simulink model "AFCSModel"  (R2025b)
settings: Solver=ode4  StartTime=0.0  StopTime=200  FixedStep=0.01  RelTol=1e-3  EnableMultiTasking=on
values from neighbouring files (symbols this model uses):
  AD = [0.05526	0.05526	0.05568	0.05804	0.06460	0.08210 ... (first row only)    [AirCraftData.m]
  Alpha0 = [0.143	0.143	0.122	-0.267	-0.627	0.120 ... (first row only)    [AirCraftData.m]
  alt = 1284.73    [Start.m]    (also in drl_simplified_dynamics.m)
  CA = 3.451    [AirCraftData.m]    (also in AircraftTrim.m)
  CDmin = [0.03799	0.03799	0.03799	0.03799	0.03904	0.04277 ... (first row only)    [AirCraftData.m]
  CLAlpha = [0.1012	0.1021	0.1033	0.1051	0.1079	0.0976 ... (first row only)    [AirCraftData.m]
  Clbt0 = [-0.00147	-0.00148	-0.00149	-0.00153	-0.00158	-0.00171 ... (first row only)    [AirCraftData.m]
  Clbtaf = [0	0	0	0	0	0;0	 0	0	0	0	0]    [AirCraftData.m]
  ClDelA = [-0.003110	-0.003065	-0.003040	-0.003036	-0.003052	-0.003088 ... (first row only)    [AirCraftData.m]
  CLDelE = [0.00653	0.00668	0.00690	0.00724	0.00772	0.00846 ... (first row only)    [AirCraftData.m]
  ClDelR = [0.000584	0.000605	0.000638	0.000686	0.000760	0.000877 ... (first row only)    [AirCraftData.m]
  CLDM = [0.244	0.244	0.244	0.244	0.244	0.244 ... (first row only)    [AirCraftData.m]
  Clp0 = [-0.5510 	-0.5610 	-0.5767 	-0.6005 	-0.6224 	-0.6763 ... (first row only)    [AirCraftData.m]
  ClpAf = [0,0,0,0,0,0;0,0,0,0,0,0]    [AirCraftData.m]
  Clr0 = [0.1308 	0.1339 	0.1383 	0.1474 	0.1601 	0.1738 ... (first row only)    [AirCraftData.m]
  ClrAf = [0,0,0,0,0,0;0,0,0,0,0,0]    [AirCraftData.m]
  Cm0 = [0.2014	0.2017	0.2034	0.2083	0.2207	0.2475 ... (first row only)    [AirCraftData.m]
  CmAfdot = [-11.5890 	-12.0169 	-12.7558 	-13.8010 	-15.2088 	-16.2278 ... (first row only)    [AirCraftData.m]
  CmCl = [-0.3454	-0.3441	-0.3427	-0.3412	-0.3396	-0.3379 ... (first row only)    [AirCraftData.m]
  CmDelE = [-0.03554	-0.03651	-0.03802	-0.04028	-0.04365	-0.04798 ... (first row only)    [AirCraftData.m]
  Cmq0 = [-42.0260 	-42.2665 	-42.9499 	-44.8315 	-45.5877 	-46.0842 ... (first row only)    [AirCraftData.m]
  CN1A0 = [0.0740	0.0662	0.0605	0.0552	0.0554 ... (first row only)    [AirCraftData.m]
  Cnbt0 = [0.00180	0.00183	0.00187	0.00192	0.00200	0.00207 ... (first row only)    [AirCraftData.m]
  Cnbtaf = [-0.000030 	-0.000031 	-0.000031 	-0.000032 	-0.000033 	-0.000035 ... (first row only)    [AirCraftData.m]
  CnDelA0 = [-0.000180	-0.000178	-0.000176	-0.000176	-0.000177	-0.000179 ... (first row only)    [AirCraftData.m]
  CnDelAAf = [0	 0	0	0	0	0;0	 0	0	0	0	0]    [AirCraftData.m]
  CnDelR = [-0.002214	-0.002274	-0.002367	-0.002505	-0.002712	-0.003039 ... (first row only)    [AirCraftData.m]
  Cnp0 = [0.0521 	0.0532 	0.0571 	0.0601 	0.0636 	0.0664 ... (first row only)    [AirCraftData.m]
  CnpAf = [0,0,0,0,0,0;0,0,0,0,0,0]    [AirCraftData.m]
  Cnr = [-0.1810 	-0.1832 	-0.1855 	-0.1892 	-0.1933 	-0.1973 ... (first row only)    [AirCraftData.m]
  Cxh_Slip = [0.0000, 0.0045, 0.0089, 0.0132, 0.0174 ... (first row only)    [AirCraftData.m]
  Cybeta0 = [-0.01783	-0.01790	-0.01804	-0.01824	-0.01851	-0.01884 ... (first row only)    [AirCraftData.m]
  Cybtaf = [0 0 0 0 0 0;0 0 0 0 0 0]    [AirCraftData.m]
  CyDelA = [0.000287	0.000295	0.000307	0.000325	0.000351	0.000394 ... (first row only)    [AirCraftData.m]
  CyDelR = [0.004946	0.005035	0.005316	0.005791	0.006458	0.007318 ... (first row only)    [AirCraftData.m]
  Cyh_Slip = [0.0000, -0.0248, -0.0519, -0.0813, -0.1130 ... (first row only)    [AirCraftData.m]
  ETA_data = [0.729 0.727 0.72 0.71 0.877 0.858 0.855 0.853 0.857 0.862 0.87 0.796 ... (330 elements, 11x5x6)]    [ETA_data.mat]
  eul_0 = [0/57.3 0/57.3 0/57.3]    [AircraftTrim.m]
  F = A(:, 1)    [drl_simplified_dynamics.m]    (also in func_DrawAircraftModel.m = [         1,  2,  3,  1;         1,  3,  4,  1;         1,  )
  flap = 0    [AircraftTrim.m]
  inertia = [  Ix      Iy     Iz  Ixz]    [AircraftTrim.m]
  Initi_Heading = 15.95*pi/180    (= 0.278380015693)    [Start.m]
  Initi_Lati = 32.6261    [Start.m]
  Initi_Longi = 103.5940    (= 103.594)    [Start.m]
  mass = 54000    [Start.m]    (also in drl_simplified_dynamics.m)
  op = evalin('base', 'op')    [drl_simplified_dynamics.m]
  q = func_GreatCircleForward(start_lat, start_lon, leg_bearing, local_s)    [system_model_update.m]
  r = r1 + r2    [drl_piecewise_reward.m]    (also in drl_reward_function.m)
  RNPAR_FlightPlan = JiuZhaiHuangLong_RNPAR_FlightPlan    [Manuscript_RNPAR_FlightPlan.m]
  Vab_0 = [Vt 0 0]    [AircraftTrim.m]
  Vt = 80    [Start.m]    (also in drl_simplified_dynamics.m; setup_afcs_system_model_test.m)
  wind_direction = 0    [Start.m]
  wind_type = 2    [Start.m]
  Wxyz_0 = [0 0 0]    [AircraftTrim.m]
  X = 1.06    [AircraftTrim.m]
  xme_0 = [0 0 -alt]    [AircraftTrim.m]
  Y = 1.177    [AircraftTrim.m]
undefined symbols (not defined in the file or in its folder): func_SystemModelMonitorBlock, Light, MIL, slselsubs, thrust_data
libraries: simulink_extras x4, aerolibatmos2 x3, aerolibconvert2 x3, aerolibwind2 x3, sharedutil x2, aerolibobsolete x1
(part 2 of 3)

== system AFCSModel/Plane&Actuator/PlaneModel/Aero Moment ==
  note: L
  note: M
  note: N
  V Alpha Beta : Inport
  QS : Inport  Port=2
  delta_a delta_e delta_r : Inport  Port=3
  p q r : Inport  Port=4
  delta_p : Inport  Port=5
  Thrust : Inport  Port=6
  delta_flap : Inport  Port=7
  Calculate Roll Moment L : Subsystem
  Calculate Yaw Moment N : Subsystem
  Calculate pitch Moment M : Subsystem
  Mux2 : Mux  Inputs=3
  Ma_b : Outport
  wires:
  Mux2/1 -> Ma_b/1
  QS/1 -> Calculate Roll Moment L/2(QS), Calculate pitch Moment M/1(QS), Calculate Yaw Moment N/2(QS)
  V Alpha Beta/1 -> Calculate Roll Moment L/1(V Alpha Beta), Calculate pitch Moment M/2(V alpha beta), Calculate Yaw Moment N/1(V Alpha Beta)
  delta_p/1 -> Calculate pitch Moment M/3(delta_p), Calculate Roll Moment L/5(delta_p), Calculate Yaw Moment N/5(delta_p)
  delta_a delta_e delta_r/1 -> Calculate Roll Moment L/3(delta_a delta_e delta_r), Calculate pitch Moment M/4(delta_a delta_e delta_r), Calculate Yaw Moment N/3(delta_a delta_e delta_r)
  p q r/1 -> Calculate Roll Moment L/4(p q r), Calculate pitch Moment M/5(p q r), Calculate Yaw Moment N/4(p q r)
  Calculate pitch Moment M/1(M) -> Mux2/2
  Calculate Roll Moment L/1(L) -> Mux2/1
  Calculate Yaw Moment N/1(N) -> Mux2/3
  Thrust/1 -> Calculate pitch Moment M/6(Thrust), Calculate Roll Moment L/6(Thrust)
  delta_flap/1 -> Calculate Roll Moment L/7(delta_flap), Calculate pitch Moment M/7(delta_flap), Calculate Yaw Moment N/6(delta_flap)

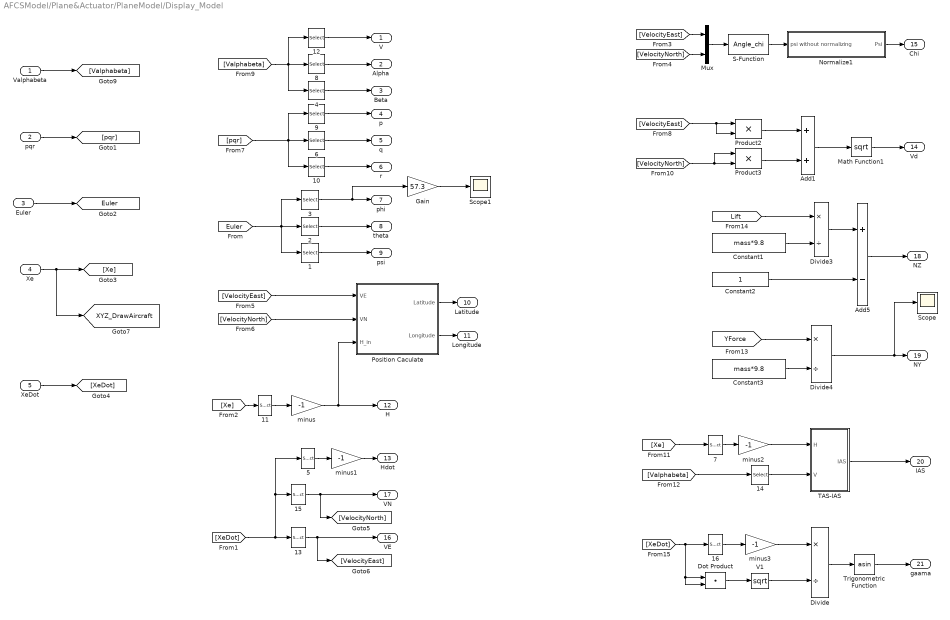
== system AFCSModel/Plane&Actuator/PlaneModel/Display_Model ==
  Valphabeta : Inport
  pqr : Inport  Port=2
  Euler : Inport  Port=3
  Xe : Inport  Port=4
  XeDot : Inport  Port=5
  {1,4..5,7,10..11,16} (7 alike) : Selector  InputPortWidth=3  IndexOptions=Index vector (dialog)  Indices=3  OutputSizes=[(-2)]
  {3,9,12,14..15} (5 alike) : Selector  InputPortWidth=3  IndexOptions=Index vector (dialog)  Indices=1  OutputSizes=[(-2)]
  {2,6,8,13} (4 alike) : Selector  InputPortWidth=3  IndexOptions=Index vector (dialog)  Indices=2  OutputSizes=[(-2)]
  Add1 : Sum
  Add5 : Sum  Inputs=+-
  Constant1 : Constant  Value=mass*9.8
  Constant2 : Constant
  Constant3 : Constant  Value=mass*9.8
  Divide : Product  Inputs=*/
  Divide3 : Product  Inputs=*/
  Divide4 : Product  Inputs=*/
  Dot Product : DotProduct  SaturateOnIntegerOverflow=on  InputSameDT=off  OutDataTypeStr=Inherit: Inherit via internal rule
  Gain : Gain  Gain=57.3
  Math Function1 : Math  Operator=sqrt  SignedPower=on
  Mux : Mux  Inputs=2
  Normalize1 : Subsystem
  Position Caculate : Subsystem
  Product2 : Product  RndMeth=Zero
  Product3 : Product  RndMeth=Zero
  S-Function : S-Function  FunctionName=Angle_chi  SFunctionDeploymentMode=off  EnableBusSupport=off
  Scope : Scope
      settings: ActiveDisplayYMinimum=-0.01745  ActiveDisplayYMaximum=0.03101  DataLoggingVariableName=ScopeData3
  Scope1 : Scope
      settings: ActiveDisplayYMinimum=-1.2868572992970082  ActiveDisplayYMaximum=11.581951961084815
  TAS-IAS : Subsystem
  Trigonometric Function : Trigonometry  Operator=asin
  V1 : Math  Operator=sqrt  SignedPower=on
  minus{,1..3} (4 alike) : Gain  Gain=-1
  V : Outport
  Alpha : Outport  Port=2
  Beta : Outport  Port=3
  p : Outport  Port=4
  q : Outport  Port=5
  r : Outport  Port=6
  phi : Outport  Port=7
  theta : Outport  Port=8
  psi : Outport  Port=9
  Latitude : Outport  Port=10
  Longitude : Outport  Port=11
  H : Outport  Port=12
  Hdot : Outport  Port=13
  Vd : Outport  Port=14
  Chi : Outport  Port=15
  VE : Outport  Port=16
  VN : Outport  Port=17
  NZ : Outport  Port=18
  NY : Outport  Port=19
  IAS : Outport  Port=20
  gaama : Outport  Port=21
  tag scope: Euler=global, XYZ_DrawAircraft=global
  wires:
  [Xe] -> 11/1
  11/1 -> minus/1
  [pqr] -> 6/1, 9/1, 10/1
  [Euler] -> 2/1, 3/1, 1/1
  [Valphabeta] -> 8/1, 12/1, 4/1
  12/1 -> V/1
  Valphabeta/1 -> [Valphabeta]
  pqr/1 -> [pqr]
  Euler/1 -> [Euler]
  Xe/1 -> [XYZ_DrawAircraft], [Xe]
  [XeDot] -> 15/1, 5/1, 13/1
  5/1 -> minus1/1
  13/1 -> [VelocityEast], VE/1
  minus1/1 -> Hdot/1
  XeDot/1 -> [XeDot]
  15/1 -> [VelocityNorth], VN/1
  S-Function/1 -> Normalize1/1(psi without normalizing)
  Normalize1/1(Psi) -> Chi/1
  Mux/1 -> S-Function/1
  [VelocityEast] -> Mux/1
  [VelocityNorth] -> Mux/2
  [VelocityEast] -> Position Caculate/1(VE)
  [VelocityNorth] -> Position Caculate/2(VN)
  Position Caculate/1(Latitude) -> Latitude/1
  Position Caculate/2(Longitude) -> Longitude/1
  Product2/1 -> Add1/1
  Product3/1 -> Add1/2
  Math Function1/1 -> Vd/1
  Add1/1 -> Math Function1/1
  [VelocityNorth] -> Product3/1, Product3/2
  [VelocityEast] -> Product2/2, Product2/1
  [Xe] -> 7/1
  7/1 -> minus2/1
  minus2/1 -> TAS-IAS/1(H)
  minus/1 -> Position Caculate/3(H_in), H/1
  [Valphabeta] -> 14/1
  14/1 -> TAS-IAS/2(V)
  TAS-IAS/1(IAS) -> IAS/1
  Divide4/1 -> Scope/1, NY/1
  Constant3/1 -> Divide4/2
  [YForce] -> Divide4/1
  [Lift] -> Divide3/1
  Constant1/1 -> Divide3/2
  Divide3/1 -> Add5/1
  Constant2/1 -> Add5/2
  Add5/1 -> NZ/1
  1/1 -> psi/1
  2/1 -> theta/1
  3/1 -> Gain/1, phi/1
  10/1 -> r/1
  6/1 -> q/1
  9/1 -> p/1
  4/1 -> Beta/1
  8/1 -> Alpha/1
  Trigonometric Function/1 -> gaama/1
  Divide/1 -> Trigonometric Function/1
  16/1 -> minus3/1
  [XeDot] -> Dot Product/2, Dot Product/1, 16/1
  Dot Product/1 -> V1/1
  minus3/1 -> Divide/1
  V1/1 -> Divide/2
  Gain/1 -> Scope1/1

== system AFCSModel/Plane&Actuator/PlaneModel/Engine ==
  Alt : Inport
  V : Inport  Port=2
  delta_p : Inport  Port=3
  Calculate Force : Lookup_n-D  NumberOfTableDimensions=3  BreakpointsForDimension1=[0,1000,2000,3000,4000,5000,6000,7000,8000,9000,10000]  BreakpointsForDimension2=[50,100,150,175,200]  BreakpointsForDimension3=[0.2,0.4,0.6,0.7,0.85,1,1.04]  BreakpointsForDimension5=slselsubs({[1:3], [1:3], [1:3], [1:3], [1:3], [1:3], [1:3], [1:3], [1:3], [1:3], [1:3], [1:3], [1:3], [1:3], [1:3], [1:3], [1:3], [1:3], [1:3], [1:3], [1:3], [1:3], [1:3], [1:3], [1:3], [1:3]}, 1)  BreakpointsForDimension6=slselsubs({[1:3], [1:3], [1:3], [1:3], [1:3], [1:3], [1:3], [1:3], [1:3], [1:3], [1:3], [1:3], [1:3], [1:3], [1:3], [1:3], [1:3], [1:3], [1:3], [1:3], [1:3], [1:3], [1:3], [1:3], [1:3], [1:3]}, 2)  BreakpointsForDimension7=slselsubs({[1:3], [1:3], [1:3], [1:3], [1:3], [1:3], [1:3], [1:3], [1:3], [1:3], [1:3], [1:3], [1:3], [1:3], [1:3], [1:3], [1:3], [1:3], [1:3], [1:3], [1:3], [1:3], [1:3], [1:3], [1:3], [1:3]}, 3)  BreakpointsForDimension8=slselsubs({[1:3], [1:3], [1:3], [1:3], [1:3], [1:3], [1:3], [1:3], [1:3], [1:3], [1:3], [1:3], [1:3], [1:3], [1:3], [1:3], [1:3], [1:3], [1:3], [1:3], [1:3], [1:3], [1:3], [1:3], [1:3], [1:3]}, 4)  BreakpointsForDimension9=slselsubs({[1:3], [1:3], [1:3], [1:3], [1:3], [1:3], [1:3], [1:3], [1:3], [1:3], [1:3], [1:3], [1:3], [1:3], [1:3], [1:3], [1:3], [1:3], [1:3], [1:3], [1:3], [1:3], [1:3], [1:3], [1:3], [1:3]}, 5)  BreakpointsForDimension10=slselsubs({[1:3], [1:3], [1:3], [1:3], [1:3], [1:3], [1:3], [1:3], [1:3], [1:3], [1:3], [1:3], [1:3], [1:3], [1:3], [1:3], [1:3], [1:3], [1:3], [1:3], [1:3], [1:3], [1:3], [1:3], [1:3], [1:3]}, 6)  BreakpointsForDimension11=slselsubs({[1:3], [1:3], [1:3], [1:3], [1:3], [1:3], [1:3], [1:3], [1:3], [1:3], [1:3], [1:3], [1:3], [1:3], [1:3], [1:3], [1:3], [1:3], [1:3], [1:3], [1:3], [1:3], [1:3], [1:3], [1:3], [1:3]}, 7)  BreakpointsForDimension12=slselsubs({[1:3], [1:3], [1:3], [1:3], [1:3], [1:3], [1:3], [1:3], [1:3], [1:3], [1:3], [1:3], [1:3], [1:3], [1:3], [1:3], [1:3], [1:3], [1:3], [1:3], [1:3], [1:3], [1:3], [1:3], [1:3], [1:3]}, 8)  BreakpointsForDimension13=slselsubs({[1:3], [1:3], [1:3], [1:3], [1:3], [1:3], [1:3], [1:3], [1:3], [1:3], [1:3], [1:3], [1:3], [1:3], [1:3], [1:3], [1:3], [1:3], [1:3], [1:3], [1:3], [1:3], [1:3], [1:3], [1:3], [1:3]}, 9)  BreakpointsForDimension14=slselsubs({[1:3], [1:3], [1:3], [1:3], [1:3], [1:3], [1:3], [1:3], [1:3], [1:3], [1:3], [1:3], [1:3], [1:3], [1:3], [1:3], [1:3], [1:3], [1:3], [1:3], [1:3], [1:3], [1:3], [1:3], [1:3], [1:3]}, 10)  BreakpointsForDimension15=slselsubs({[1:3], [1:3], [1:3], [1:3], [1:3], [1:3], [1:3], [1:3], [1:3], [1:3], [1:3], [1:3], [1:3], [1:3], [1:3], [1:3], [1:3], [1:3], [1:3], [1:3], [1:3], [1:3], [1:3], [1:3], [1:3], [1:3]}, 11)  BreakpointsForDimension16=slselsubs({[1:3], [1:3], [1:3], [1:3], [1:3], [1:3], [1:3], [1:3], [1:3], [1:3], [1:3], [1:3], [1:3], [1:3], [1:3], [1:3], [1:3], [1:3], [1:3], [1:3], [1:3], [1:3], [1:3], [1:3], [1:3], [1:3]}, 12)  BreakpointsForDimension17=slselsubs({[1:3], [1:3], [1:3], [1:3], [1:3], [1:3], [1:3], [1:3], [1:3], [1:3], [1:3], [1:3], [1:3], [1:3], [1:3], [1:3], [1:3], [1:3], [1:3], [1:3], [1:3], [1:3], [1:3], [1:3], [1:3], [1:3]}, 13)  BreakpointsForDimension18=slselsubs({[1:3], [1:3], [1:3], [1:3], [1:3], [1:3], [1:3], [1:3], [1:3], [1:3], [1:3], [1:3], [1:3], [1:3], [1:3], [1:3], [1:3], [1:3], [1:3], [1:3], [1:3], [1:3], [1:3], [1:3], [1:3], [1:3]}, 14)  BreakpointsForDimension19=slselsubs({[1:3], [1:3], [1:3], [1:3], [1:3], [1:3], [1:3], [1:3], [1:3], [1:3], [1:3], [1:3], [1:3], [1:3], [1:3], [1:3], [1:3], [1:3], [1:3], [1:3], [1:3], [1:3], [1:3], [1:3], [1:3], [1:3]}, 15)  BreakpointsForDimension20=slselsubs({[1:3], [1:3], [1:3], [1:3], [1:3], [1:3], [1:3], [1:3], [1:3], [1:3], [1:3], [1:3], [1:3], [1:3], [1:3], [1:3], [1:3], [1:3], [1:3], [1:3], [1:3], [1:3], [1:3], [1:3], [1:3], [1:3]}, 16)  BreakpointsForDimension21=slselsubs({[1:3], [1:3], [1:3], [1:3], [1:3], [1:3], [1:3], [1:3], [1:3], [1:3], [1:3], [1:3], [1:3], [1:3], [1:3], [1:3], [1:3], [1:3], [1:3], [1:3], [1:3], [1:3], [1:3], [1:3], [1:3], [1:3]}, 17)  BreakpointsForDimension22=slselsubs({[1:3], [1:3], [1:3], [1:3], [1:3], [1:3], [1:3], [1:3], [1:3], [1:3], [1:3], [1:3], [1:3], [1:3], [1:3], [1:3], [1:3], [1:3], [1:3], [1:3], [1:3], [1:3], [1:3], [1:3], [1:3], [1:3]}, 18)  BreakpointsForDimension23=slselsubs({[1:3], [1:3], [1:3], [1:3], [1:3], [1:3], [1:3], [1:3], [1:3], [1:3], [1:3], [1:3], [1:3], [1:3], [1:3], [1:3], [1:3], [1:3], [1:3], [1:3], [1:3], [1:3], [1:3], [1:3], [1:3], [1:3]}, 19)  BreakpointsForDimension24=slselsubs({[1:3], [1:3], [1:3], [1:3], [1:3], [1:3], [1:3], [1:3], [1:3], [1:3], [1:3], [1:3], [1:3], [1:3], [1:3], [1:3], [1:3], [1:3], [1:3], [1:3], [1:3], [1:3], [1:3], [1:3], [1:3], [1:3]}, 20)  BreakpointsForDimension25=slselsubs({[1:3], [1:3], [1:3], [1:3], [1:3], [1:3], [1:3], [1:3], [1:3], [1:3], [1:3], [1:3], [1:3], [1:3], [1:3], [1:3], [1:3], [1:3], [1:3], [1:3], [1:3], [1:3], [1:3], [1:3], [1:3], [1:3]}, 21)  BreakpointsForDimension26=slselsubs({[1:3], [1:3], [1:3], [1:3], [1:3], [1:3], [1:3], [1:3], [1:3], [1:3], [1:3], [1:3], [1:3], [1:3], [1:3], [1:3], [1:3], [1:3], [1:3], [1:3], [1:3], [1:3], [1:3], [1:3], [1:3], [1:3]}, 22)  BreakpointsForDimension27=slselsubs({[1:3], [1:3], [1:3], [1:3], [1:3], [1:3], [1:3], [1:3], [1:3], [1:3], [1:3], [1:3], [1:3], [1:3], [1:3], [1:3], [1:3], [1:3], [1:3], [1:3], [1:3], [1:3], [1:3], [1:3], [1:3], [1:3]}, 23)  BreakpointsForDimension28=slselsubs({[1:3], [1:3], [1:3], [1:3], [1:3], [1:3], [1:3], [1:3], [1:3], [1:3], [1:3], [1:3], [1:3], [1:3], [1:3], [1:3], [1:3], [1:3], [1:3], [1:3], [1:3], [1:3], [1:3], [1:3], [1:3], [1:3]}, 24)  BreakpointsForDimension29=slselsubs({[1:3], [1:3], [1:3], [1:3], [1:3], [1:3], [1:3], [1:3], [1:3], [1:3], [1:3], [1:3], [1:3], [1:3], [1:3], [1:3], [1:3], [1:3], [1:3], [1:3], [1:3], [1:3], [1:3], [1:3], [1:3], [1:3]}, 25)  BreakpointsForDimension30=slselsubs({[1:3], [1:3], [1:3], [1:3], [1:3], [1:3], [1:3], [1:3], [1:3], [1:3], [1:3], [1:3], [1:3], [1:3], [1:3], [1:3], [1:3], [1:3], [1:3], [1:3], [1:3], [1:3], [1:3], [1:3], [1:3], [1:3]}, 26)  Table=thrust_data  InterpMethod=Cubic spline  ExtrapMethod=Cubic spline
      settings: InputPortMap=u0,u1,u2
  Thrust : Outport
  wires:
  Calculate Force/1 -> Thrust/1
  delta_p/1 -> Calculate Force/3
  Alt/1 -> Calculate Force/1
  V/1 -> Calculate Force/2

== system AFCSModel/Plane&Actuator/PlaneModel/ISA ==
  note: V
  note: V^2
  V : Inport
  Alt : Inport  Port=2
  Constant2 : Constant  Value=0.5
  Divide : Product  Inputs=/*
  ISA Atmosphere Model : aerolibatmos2/ISA Atmosphere Model  useExtended=off  action=Warning  custom=off  viscosityOut=off  g=9.80665  gamma=1.4  R=287.0531  L=0.0065  h_trop=11000  h_strat=20000  rho0=1.225  P0=101325  T0=288.15  h0=0  S=110.4  Tref=273.15  muref=1.716e-5
  Product : Product  Inputs=3  RndMeth=Zero
  Product2 : Product  RndMeth=Zero
  Scope1 : Scope
  Scope2 : Scope
      settings: DataLoggingVariableName=ScopeData2
  To Workspace : ToWorkspace  VariableName=Rou  SampleTime=-1
  Qs : Outport
  tag scope: Alt=global, Ma=global
  wires:
  ISA Atmosphere Model/4 -> To Workspace/1, Product/1
  Alt/1 -> ISA Atmosphere Model/1, [Alt]
  ISA Atmosphere Model/1 -> Scope2/1
  ISA Atmosphere Model/3 -> Scope1/1
  Product/1 -> Qs/1
  Divide/1 -> [Ma]
  ISA Atmosphere Model/2 -> Divide/1
  Product2/1 -> Product/3
  Constant2/1 -> Product/2
  V/1 -> Divide/2, Product2/1, Product2/2

== system AFCSModel/Plane&Actuator/PlaneModel/RusPlane ==
  Force : Inport
  Moment : Inport  Port=2
  AV Alpha Beta : Subsystem
  AV Alpha Beta_Trans : Subsystem
  BWxyz2 : Integrator  InitialCondition=op.States(2).x
  Calculate DCM & Euler Angles : Subsystem  AncestorBlock=aerolib6dofsys/DCM & Euler Angles (Euler)  mask(DCM & Euler Angles (Euler)){}
  Constant1 : Constant  Value=inertia  OutDataTypeStr=Inherit: Inherit via back propagation
  Constant2 : Constant  Value=mass  OutDataTypeStr=Inherit: Inherit via back propagation
  Product : Product  Inputs=*/  SaturateOnIntegerOverflow=on  OutDataTypeStr=Inherit: Same as first input
  Subsystem : Subsystem
  Subsystem1 : Subsystem
  Sum : Sum  Inputs=|++  SaturateOnIntegerOverflow=on
  Vbxw : sharedutil/3x3 Cross Product  aMode=aMode
      settings: LibrarySourceBlock=aerolibutil/3x3 Cross Product
  xe,ye,ze : Integrator  InitialCondition=op.States(4).x
  V alpha beta : Outport
  p q r : Outport  Port=2
  Euler : Outport  Port=3
  Xe : Outport  Port=4
  XeDot : Outport  Port=5
  tag scope: Plane_uvw=global
  wires:
  Constant1/1 -> Subsystem/3(inertia Ix Iy Iz Ixz)
  Product/1 -> Sum/1
  Sum/1 -> AV Alpha Beta/1(udot vdot wdot)
  Vbxw/1 -> Sum/2
  Constant2/1 -> Product/2
  BWxyz2/1 -> Calculate DCM & Euler Angles/1("Wxyz "), p q r/1, Vbxw/2, Subsystem/2(pqr)  "pqr"
  Subsystem1/1(Xedot Yedot Zedot) -> XeDot/1, xe,ye,ze/1
  Force/1 -> Product/1  "Force"
  xe,ye,ze/1 -> Xe/1  "Xe"
  Calculate DCM & Euler Angles/1(Euler) -> Euler/1, Subsystem1/2(Euler phi theta psi)  "Eular"
  AV Alpha Beta/2(u v w in) -> Vbxw/1, [Plane_uvw], Subsystem1/1("U V W ")
  AV Alpha Beta/1(V alpha beta) -> AV Alpha Beta_Trans/1(V alpha beta input)
  Subsystem/1(pdot qdot rdot) -> BWxyz2/1
  Moment/1 -> Subsystem/1(Moment L M N)  "Moment"
  AV Alpha Beta_Trans/1(Valphabeta) -> V alpha beta/1

== system AFCSModel/RNP AR Approach Guidance/L1GuidanceVersion1/Subsystem ==
  YZ : Inport
  Lfw : Inport  Port=2
  eta1 : Inport  Port=3
  R_turn : Inport  Port=4
  turnDir : Inport  Port=5
  legType : Inport  Port=6
  Divide : Product  Inputs=*/
  Gain : Gain  Gain=-1
  Plus : Sum
  Scope : Scope
      settings: ActiveDisplayYMinimum=-1  ActiveDisplayYMaximum=1  DataLoggingVariableName=ScopeData9
  Scope1 : Scope
      settings: ActiveDisplayYMinimum=-1  ActiveDisplayYMaximum=1  DataLoggingVariableName=ScopeData10
  Square : Math  Operator=square
  Square1 : Math  Operator=square
  caculateL1 : Sqrt
  eta2TF : Trigonometry  Operator=atan
  etaTF : Sum
  L1 : Outport
  eta : Outport  Port=2
  wires:
  Square1/1 -> Plus/2
  Square/1 -> Plus/1
  Plus/1 -> caculateL1/1
  YZ/1 -> Square/1, Divide/1
  Lfw/1 -> Square1/1, Divide/2
  Divide/1 -> eta2TF/1
  eta1/1 -> Gain/1
  eta2TF/1 -> etaTF/2, Scope1/1
  etaTF/1 -> eta/1
  Gain/1 -> Scope/1, etaTF/1
  caculateL1/1 -> L1/1

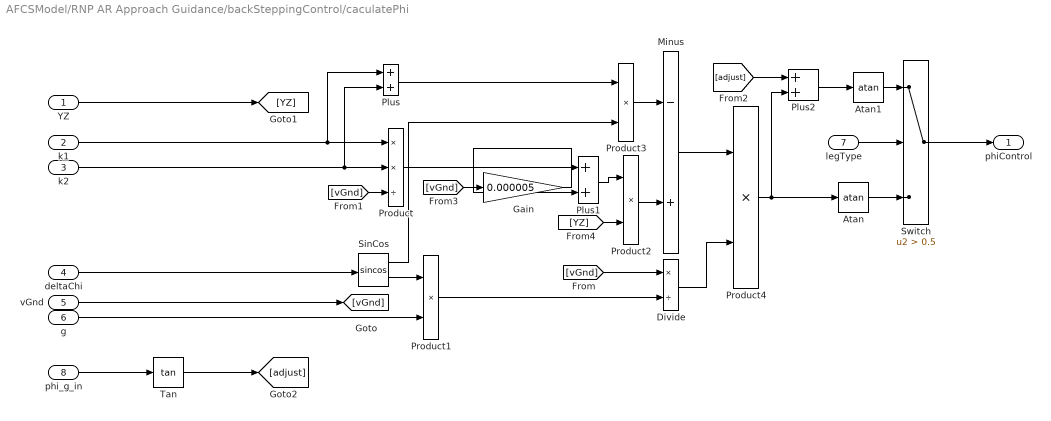
== system AFCSModel/RNP AR Approach Guidance/backSteppingControl/caculatePhi ==
  YZ : Inport
  k1 : Inport  Port=2
  k2 : Inport  Port=3
  deltaChi : Inport  Port=4
  vGnd : Inport  Port=5
  g : Inport  Port=6
  legType : Inport  Port=7
  phi_g_in : Inport  Port=8
  Atan : Trigonometry  Operator=atan
  Atan1 : Trigonometry  Operator=atan
  Divide : Product  Inputs=*/
  Gain : Gain  Gain=0.000005
  Minus : Sum  Inputs=-+
  Plus : Sum
  Plus1 : Sum
  Plus2 : Sum
  Product : Product  Inputs=**/
  Product{1..4} (4 alike) : Product
  SinCos : Trigonometry  Operator=sincos
  Switch : Switch  Criteria=u2 > Threshold  Threshold=0.5  SaturateOnIntegerOverflow=off  InputSameDT=off
  Tan : Trigonometry  Operator=tan
  phiControl : Outport
  wires:
  [vGnd] -> Divide/1
  Product/1 -> Plus1/1
  Product2/1 -> Minus/2
  g/1 -> Product1/2
  k1/1 -> Product/1, Plus/1
  k2/1 -> Product/2, Plus/2
  [vGnd] -> Product/3
  SinCos/2 -> Product1/1
  deltaChi/1 -> SinCos/1
  Plus/1 -> Product3/1
  Plus1/1 -> Product2/1
  Product1/1 -> Divide/2
  Product3/1 -> Minus/1
  SinCos/1 -> Product3/2
  [YZ] -> Product2/2
  YZ/1 -> [YZ]
  vGnd/1 -> [vGnd]
  Minus/1 -> Product4/1
  Divide/1 -> Product4/2
  Product4/1 -> Atan/1, Plus2/2
  Atan/1 -> Switch/3
  legType/1 -> Switch/2
  Switch/1 -> phiControl/1
  [adjust] -> Plus2/1
  Plus2/1 -> Atan1/1
  Atan1/1 -> Switch/1
  phi_g_in/1 -> Tan/1
  Tan/1 -> [adjust]
  [vGnd] -> Gain/1
  Gain/1 -> Plus1/2

== system AFCSModel/RNP AR Approach Guidance/backSteppingControlTanh/Subsystem ==
  z2 : Inport
  z1 : Inport  Port=2
  f1 : Inport  Port=3
  deltaChi : Inport  Port=4
  vGnd : Inport  Port=5
  phi_g_in : Inport  Port=6
  legType : Inport  Port=7
  Atan : Trigonometry  Operator=atan
  Atan1 : Trigonometry  Operator=atan
  Constant : Constant  Value=9.81
  Product{,1..3} (4 alike) : Product
  SinCos : Trigonometry  Operator=sincos
  Sum : Sum  Inputs=|++
  Switch : Switch  Criteria=u2 > Threshold  Threshold=0.5  SaturateOnIntegerOverflow=off  InputSameDT=off
  Tan : Trigonometry  Operator=tan
  caculateMultiplier : Product  Inputs=/*
  caculateUfb : Sum  Inputs=-+-
  k1 : Gain  Gain=0.25
  k2 : Gain  Gain=0.25
  k3 : Gain  Gain=0.25
  phiCmd : Outport
  wires:
  Constant/1 -> Product2/2
  SinCos/2 -> Product2/1
  Product/1 -> caculateUfb/2
  f1/1 -> Product/2, k1/1
  Product2/1 -> caculateMultiplier/1
  z2/1 -> k2/1
  Product1/1 -> caculateUfb/3
  SinCos/1 -> Product1/2
  k1/1 -> Product1/1
  k2/1 -> caculateUfb/1
  deltaChi/1 -> SinCos/1
  z1/1 -> Product/1
  Tan/1 -> Sum/1
  vGnd/1 -> caculateMultiplier/2
  phi_g_in/1 -> Tan/1
  caculateUfb/1 -> Product3/1
  caculateMultiplier/1 -> Product3/2
  Product3/1 -> Atan/1, Sum/2
  legType/1 -> Switch/2
  Atan/1 -> Switch/3
  Sum/1 -> Atan1/1
  Atan1/1 -> Switch/1
  Switch/1 -> phiCmd/1

== system AFCSModel/RNP AR Approach Guidance/backSteppingControlTanh/caculateZ1F1 ==
  YZ : Inport
  vGnd : Inport  Port=2
  Constant : Constant
  Kp : Constant  Value=0.002
  Plus : Sum  Inputs=-+
  Product : Product
  Product1 : Product
  Product2 : Product
  Square : Math  Operator=square
  Tanh : Trigonometry  Operator=tanh
  z1 : Outport
  f1 : Outport  Port=2
  wires:
  Product/1 -> Tanh/1
  Tanh/1 -> z1/1, Square/1
  YZ/1 -> Product/1
  Kp/1 -> Product1/1, Product/2
  vGnd/1 -> Product1/2
  Square/1 -> Plus/1
  Constant/1 -> Plus/2
  Plus/1 -> Product2/1
  Product1/1 -> Product2/2
  Product2/1 -> f1/1

== system AFCSModel/RNP AR Approach Guidance/backSteppingControlTanh/caculateZ2 ==
  deltaChi : Inport
  z1 : Inport  Port=2
  Plus : Sum  Inputs=+-
  Sin : Trigonometry
  k1 : Gain  Gain=0.25
  z2 : Outport
  wires:
  Sin/1 -> Plus/1
  Plus/1 -> z2/1
  k1/1 -> Plus/2
  z1/1 -> k1/1
  deltaChi/1 -> Sin/1

== system AFCSModel/RNP AR Approach Guidance/ndiControl/calculatePhi ==
  vControl : Inport
  deltaChi : Inport  Port=2
  vGnd : Inport  Port=3
  phi_g_in : Inport  Port=4
  Atan : Trigonometry  Operator=atan
  Atan1 : Trigonometry  Operator=atan
  Derivative : Derivative
  Divide : Product  Inputs=*/
  Minus : Sum  Inputs=-+
  Product : Product
  Product1 : Product
  Scope : Scope
      settings: ActiveDisplayYMinimum=-0.11968  ActiveDisplayYMaximum=0.06057  DataLoggingVariableName=ScopeData2
  SinCos : Trigonometry  Operator=sincos
  Sum : Sum  Inputs=++|
  Tan : Trigonometry  Operator=tan
  g : Constant  Value=9.81
  rfPhi : Outport
  tfPhi : Outport  Port=2
  wires:
  Atan/1 -> tfPhi/1
  Divide/1 -> Atan/1, Sum/1
  phi_g_in/1 -> Tan/1, Scope/1
  Sum/1 -> Atan1/1
  Atan1/1 -> rfPhi/1
  Tan/1 -> Sum/2
  deltaChi/1 -> SinCos/1
  Product/1 -> Divide/2
  vGnd/1 -> Derivative/1
  Derivative/1 -> Product1/1
  SinCos/1 -> Product1/2
  vControl/1 -> Minus/2
  Minus/1 -> Divide/1
  SinCos/2 -> Product/1
  g/1 -> Product/2
  Product1/1 -> Minus/1

== system AFCSModel/Wind_Model/DCM_e2b/A11 ==
  sin_cos : Inport
  Demux : Demux  Outputs=2
  Selector : Selector  InputPortWidth=6  IndexOptions=Index vector (dialog)  Indices=[4 6 ]  OutputSizes=1
  cos(theta)*cos(psi) : Product  RndMeth=Zero
  A11 : Outport
  wires:
  Demux/2 -> cos(theta)*cos(psi)/2
  Demux/1 -> cos(theta)*cos(psi)/1
  Selector/1 -> Demux/1
  cos(theta)*cos(psi)/1 -> A11/1
  sin_cos/1 -> Selector/1

== system AFCSModel/Wind_Model/DCM_e2b/A12 ==
  sin_cos : Inport
  Demux : Demux  Outputs=2
  Selector : Selector  InputPortWidth=6  IndexOptions=Index vector (dialog)  Indices=[4 5]  OutputSizes=1
  cos(theta)*sin(psi) : Product  RndMeth=Zero
  A12 : Outport
  wires:
  sin_cos/1 -> Selector/1
  cos(theta)*sin(psi)/1 -> A12/1
  Selector/1 -> Demux/1
  Demux/1 -> cos(theta)*sin(psi)/1
  Demux/2 -> cos(theta)*sin(psi)/2

== system AFCSModel/Wind_Model/DCM_e2b/A13 ==
  sin_cos : Inport
  -sin(theta) : Gain  Gain=-1
  Selector : Selector  InputPortWidth=6  IndexOptions=Index vector (dialog)  Indices=3  OutputSizes=1
  A13 : Outport
  wires:
  Selector/1 -> -sin(theta)/1
  -sin(theta)/1 -> A13/1
  sin_cos/1 -> Selector/1

== system AFCSModel/Wind_Model/DCM_e2b/A21 ==
  sin_cos : Inport
  Add : Sum  Inputs=+-
  Demux : Demux  Outputs=3
  Demux1 : Demux  Outputs=2
  Selector : Selector  InputPortWidth=6  IndexOptions=Index vector (dialog)  Indices=[1 3 6]  OutputSizes=1
  Selector1 : Selector  InputPortWidth=6  IndexOptions=Index vector (dialog)  Indices=[2 5]  OutputSizes=1
  cos(phi)*sin(psi) : Product  RndMeth=Zero
  sin(phi)*sin(theta)*cos(psi) : Product  Inputs=3  RndMeth=Zero
  A21 : Outport
  wires:
  sin_cos/1 -> Selector1/1, Selector/1
  Add/1 -> A21/1
  Selector/1 -> Demux/1
  Demux/1 -> sin(phi)*sin(theta)*cos(psi)/1
  Demux/2 -> sin(phi)*sin(theta)*cos(psi)/2
  Demux/3 -> sin(phi)*sin(theta)*cos(psi)/3
  Demux1/1 -> cos(phi)*sin(psi)/1
  Demux1/2 -> cos(phi)*sin(psi)/2
  Selector1/1 -> Demux1/1
  cos(phi)*sin(psi)/1 -> Add/2
  sin(phi)*sin(theta)*cos(psi)/1 -> Add/1

== system AFCSModel/Wind_Model/DCM_e2b/A22 ==
  sin_cos : Inport
  Add : Sum
  Demux : Demux  Outputs=3
  Demux1 : Demux  Outputs=2
  Selector : Selector  InputPortWidth=6  IndexOptions=Index vector (dialog)  Indices=[1 3 5]  OutputSizes=1
  Selector2 : Selector  InputPortWidth=6  IndexOptions=Index vector (dialog)  Indices=[2 6]  OutputSizes=1
  cos(phi)*cos(psi) : Product  RndMeth=Zero
  sin(phi)*sin(theta)*sin(psi) : Product  Inputs=3  RndMeth=Zero
  A22 : Outport
  wires:
  Demux/2 -> sin(phi)*sin(theta)*sin(psi)/2
  Demux/1 -> sin(phi)*sin(theta)*sin(psi)/1
  Selector/1 -> Demux/1
  sin_cos/1 -> Selector2/1, Selector/1
  Demux/3 -> sin(phi)*sin(theta)*sin(psi)/3
  Demux1/1 -> cos(phi)*cos(psi)/1
  Demux1/2 -> cos(phi)*cos(psi)/2
  Selector2/1 -> Demux1/1
  cos(phi)*cos(psi)/1 -> Add/2
  Add/1 -> A22/1
  sin(phi)*sin(theta)*sin(psi)/1 -> Add/1

== system AFCSModel/Wind_Model/DCM_e2b/A23 ==
  sin_cos : Inport
  Demux : Demux  Outputs=2
  Selector : Selector  InputPortWidth=6  IndexOptions=Index vector (dialog)  Indices=[1 4]  OutputSizes=1
  sin(phi)*cos(theta) : Product  RndMeth=Zero
  A23 : Outport
  wires:
  sin_cos/1 -> Selector/1
  sin(phi)*cos(theta)/1 -> A23/1
  Selector/1 -> Demux/1
  Demux/1 -> sin(phi)*cos(theta)/1
  Demux/2 -> sin(phi)*cos(theta)/2

== system AFCSModel/Wind_Model/DCM_e2b/A31 ==
  sin_cos : Inport
  Add : Sum
  Demux : Demux  Outputs=3
  Demux1 : Demux  Outputs=2
  Selector : Selector  InputPortWidth=6  IndexOptions=Index vector (dialog)  Indices=[2 3 6]  OutputSizes=1
  Selector1 : Selector  InputPortWidth=6  IndexOptions=Index vector (dialog)  Indices=[1 5]  OutputSizes=1
  cos(phi)*sin(theta)*cos(psi) : Product  Inputs=3  RndMeth=Zero
  sin(phi)*sin(psi) : Product  RndMeth=Zero
  A31 : Outport
  wires:
  Demux/2 -> cos(phi)*sin(theta)*cos(psi)/2
  Demux/1 -> cos(phi)*sin(theta)*cos(psi)/1
  Selector/1 -> Demux/1
  sin_cos/1 -> Selector1/1, Selector/1
  Demux1/2 -> sin(phi)*sin(psi)/2
  Demux1/1 -> sin(phi)*sin(psi)/1
  Selector1/1 -> Demux1/1
  sin(phi)*sin(psi)/1 -> Add/2
  Demux/3 -> cos(phi)*sin(theta)*cos(psi)/3
  Add/1 -> A31/1
  cos(phi)*sin(theta)*cos(psi)/1 -> Add/1

== system AFCSModel/Wind_Model/DCM_e2b/A32 ==
  sin_cos : Inport
  Add : Sum  Inputs=+-
  Demux : Demux  Outputs=3
  Demux1 : Demux  Outputs=2
  Selector : Selector  InputPortWidth=6  IndexOptions=Index vector (dialog)  Indices=[2 3 5]  OutputSizes=1
  Selector1 : Selector  InputPortWidth=6  IndexOptions=Index vector (dialog)  Indices=[1 6]  OutputSizes=1
  cos(phi)*sin(theta)*sin(psi) : Product  Inputs=3  RndMeth=Zero
  sin(phi)*cos(psi) : Product  RndMeth=Zero
  A32 : Outport
  wires:
  Demux/2 -> cos(phi)*sin(theta)*sin(psi)/2
  Demux/1 -> cos(phi)*sin(theta)*sin(psi)/1
  Selector/1 -> Demux/1
  sin_cos/1 -> Selector1/1, Selector/1
  Demux1/2 -> sin(phi)*cos(psi)/2
  Demux1/1 -> sin(phi)*cos(psi)/1
  Selector1/1 -> Demux1/1
  sin(phi)*cos(psi)/1 -> Add/2
  Demux/3 -> cos(phi)*sin(theta)*sin(psi)/3
  Add/1 -> A32/1
  cos(phi)*sin(theta)*sin(psi)/1 -> Add/1

== system AFCSModel/Wind_Model/DCM_e2b/A33 ==
  sin_cos : Inport
  Demux : Demux  Outputs=2
  Selector : Selector  InputPortWidth=6  IndexOptions=Index vector (dialog)  Indices=[2 4]  OutputSizes=1
  cos(phi)*cos(theta) : Product  RndMeth=Zero
  A33 : Outport
  wires:
  Demux/2 -> cos(phi)*cos(theta)/2
  Demux/1 -> cos(phi)*cos(theta)/1
  Selector/1 -> Demux/1
  cos(phi)*cos(theta)/1 -> A33/1
  sin_cos/1 -> Selector/1

== system AFCSModel/Plane&Actuator/PlaneModel/Aero Force/Caculate Y ==
  note: V
  note: beta
  note: alpha
  delta_a : Inport
  delta_r : Inport  Port=2
  Qs : Inport  Port=3
  delta_p : Inport  Port=4
  " V Alpha Beta" : Inport  Port=5
  delta_flap : Inport  Port=6
  Add : Sum  Inputs=+++
  Add1 : Sum  Inputs=+-
  Cy_beta : Subsystem
  Cy_delta_a : Lookup2D  RowIndex=[0 6/57.3]  ColumnIndex=Mach_table  Table=CyDelA  SaturateOnIntegerOverflow=off  InputSameDT=off
  Cy_delta_r : Lookup2D  RowIndex=[0 6/57.3]  ColumnIndex=Mach_table  Table=CyDelR  SaturateOnIntegerOverflow=off  InputSameDT=off
  Normal force CN-alpha : Lookup2D  RowIndex=[0.4,0.7,0.85,1,1.04]  ColumnIndex=[50,75,100,150,175]  Table=CN1A0  SaturateOnIntegerOverflow=off  InputSameDT=off
  Product{1..4} (4 alike) : Product  RndMeth=Zero
  S1 : Gain  Gain=4
  S2 : Gain  Gain=121.86
  Selector1 : Selector  InputPortWidth=3  IndexOptions=Index vector (dialog)  Indices=[1]  OutputSizes=[(-2)]
  Selector2 : Selector  InputPortWidth=3  IndexOptions=Index vector (dialog)  Indices=[3]  OutputSizes=[(-2)]
  Selector3 : Selector  InputPortWidth=3  IndexOptions=Index vector (dialog)  Indices=[2]  OutputSizes=[(-2)]
  Y Force : Outport
  wires:
  [Ma] -> Cy_delta_a/2, Cy_delta_r/2, Cy_beta/1(Ma)
  Cy_delta_a/1 -> Product2/2
  Cy_delta_r/1 -> Product3/2
  Product2/1 -> Add/1
  Product3/1 -> Add/2
  Product1/1 -> Add/3
  Add/1 -> Product4/2
  delta_a/1 -> Product2/1
  Qs/1 -> Product4/1
  Product4/1 -> S2/1
  Selector2/1 -> Product1/2
  delta_r/1 -> Product3/1
  " V Alpha Beta"/1 -> Selector1/1, Selector2/1, Selector3/1
  Selector3/1 -> Cy_beta/2(alpha)
  Cy_beta/1(Cybeta) -> Add1/1
  Add1/1 -> Product1/1
  Normal force CN-alpha/1 -> S1/1
  delta_p/1 -> Normal force CN-alpha/1
  Selector1/1 -> Normal force CN-alpha/2
  S2/1 -> Y Force/1
  S1/1 -> Add1/2
  delta_flap/1 -> Cy_delta_a/1, Cy_delta_r/1, Cy_beta/3(delta_flap)

== system AFCSModel/Plane&Actuator/PlaneModel/Aero Force/Calculate  Lift ==
  note: Alpha
  note: Alpha_B
  note: V
  Qs : Inport
  " V Alpha" : Inport  Port=2
  delta_e : Inport  Port=3
  delta_p : Inport  Port=4
  Thrust : Inport  Port=5
  delta_flap : Inport  Port=6
  Add : Sum  Inputs=+++
  Caculate CL : Subsystem
  Normal force CN-alpha : Lookup2D  RowIndex=[0.4,0.7,0.85,1,1.04]  ColumnIndex=[50,75,100,150,175]  Table=CN1A0  SaturateOnIntegerOverflow=off  InputSameDT=off
  Product1 : Product  RndMeth=Zero
  S : Gain
  S1 : Gain  Gain=4
  S2 : Gain  Gain=121.86
  S3 : Gain  Gain=1.3
  Selector1 : Selector  InputPortWidth=2  IndexOptions=Index vector (dialog)  Indices=[1]  OutputSizes=[(-2)]
  Selector8 : Selector  InputPortWidth=2  IndexOptions=Index vector (dialog)  Indices=[2]  OutputSizes=[(-2)]
  SlipStream Strength B : Subsystem
  Slipstream CL : Lookup2D  RowIndex=[0,2,4,6,8,10,12,14,16 18]  ColumnIndex=[0 0.25 0.5 0.75 1]  Table=Cyh_Slip  SaturateOnIntegerOverflow=off  InputSameDT=off
  Stablizer Lift1 : Product  RndMeth=Zero
  alpha_w_deg : Subsystem
  Lift : Outport
  wires:
  Add/1 -> Product1/2
  Selector1/1 -> Normal force CN-alpha/2
  Stablizer Lift1/1 -> S1/1
  " V Alpha"/1 -> Selector8/1, Selector1/1
  Qs/1 -> Product1/1, SlipStream Strength B/2(Qs)
  Product1/1 -> S2/1
  SlipStream Strength B/1(B) -> Slipstream CL/2
  Slipstream CL/1 -> S/1
  S/1 -> Add/3
  S1/1 -> Add/2
  Selector8/1 -> Caculate CL/1(Alpha), Stablizer Lift1/1, alpha_w_deg/1(In1)
  Thrust/1 -> SlipStream Strength B/1(Thrust)
  delta_e/1 -> Caculate CL/2(delta_e)
  Caculate CL/1(CL) -> Add/1
  Normal force CN-alpha/1 -> S3/1
  delta_p/1 -> Normal force CN-alpha/1
  S2/1 -> Lift/1
  alpha_w_deg/1(Out1) -> Slipstream CL/1
  S3/1 -> Stablizer Lift1/2
  delta_flap/1 -> Caculate CL/3(delta_flap)

== system AFCSModel/Plane&Actuator/PlaneModel/Aero Force/Calculate Drag ==
  note: V
  note: Alpha
  " V Alpha" : Inport
  Thrust : Inport  Port=2
  Qs : Inport  Port=3
  delta_p : Inport  Port=4
  delta_flap : Inport  Port=5
  Add : Sum  Inputs=+++
  "Caculate CD " : Subsystem
  Normal force CN-alpha : Lookup2D  RowIndex=[0.4,0.7,0.85,1,1.04]  ColumnIndex=[50,75,100,150,175]  Table=CN1A0  SaturateOnIntegerOverflow=off  InputSameDT=off
  Product1 : Product  RndMeth=Zero
  Product2 : Product  RndMeth=Zero
  Product3 : Product  RndMeth=Zero
  S1 : Gain
  S2 : Gain  Gain=1.3
  S3 : Gain  Gain=4
  S4 : Gain  Gain=121.86
  Selector1 : Selector  InputPortWidth=2  IndexOptions=Index vector (dialog)  Indices=[1]  OutputSizes=[(-2)]
  Selector8 : Selector  InputPortWidth=2  IndexOptions=Index vector (dialog)  Indices=[2]  OutputSizes=[(-2)]
  SlipStream Strength B : Subsystem
  Slipstream CD : Lookup2D  RowIndex=[0,2,4,6,8,10,12,14,16,18]  ColumnIndex=[0,0.25,0.5,0.75,1]  Table=Cxh_Slip  SaturateOnIntegerOverflow=off  InputSameDT=off
  Trigonometric Function1 : Trigonometry
  Wing Angle : Constant  Value=4/57.3
  alpha_w : Sum
  alpha_w_deg : Subsystem
  Drag : Outport
  wires:
  SlipStream Strength B/1(B) -> Slipstream CD/2
  Slipstream CD/1 -> S1/1
  Add/1 -> Product1/1
  S1/1 -> Add/2
  " V Alpha"/1 -> Selector8/1, Selector1/1
  Thrust/1 -> SlipStream Strength B/1(Thrust)
  Qs/1 -> SlipStream Strength B/2(Qs), Product1/2
  Product1/1 -> S4/1
  "Caculate CD "/1(CD) -> Add/1
  alpha_w_deg/1(Out1) -> Slipstream CD/1
  alpha_w/1 -> "Caculate CD "/2("  Alpha_w"), alpha_w_deg/1(In1)
  Wing Angle/1 -> alpha_w/1
  Selector8/1 -> alpha_w/2, Product3/1, Trigonometric Function1/1
  Normal force CN-alpha/1 -> S2/1
  Product3/1 -> Product2/2
  Trigonometric Function1/1 -> Product2/1
  Product2/1 -> S3/1
  S3/1 -> Add/3
  delta_p/1 -> Normal force CN-alpha/1
  Selector1/1 -> Normal force CN-alpha/2
  S4/1 -> Drag/1
  S2/1 -> Product3/2
  delta_flap/1 -> "Caculate CD "/1(" delta_flap")

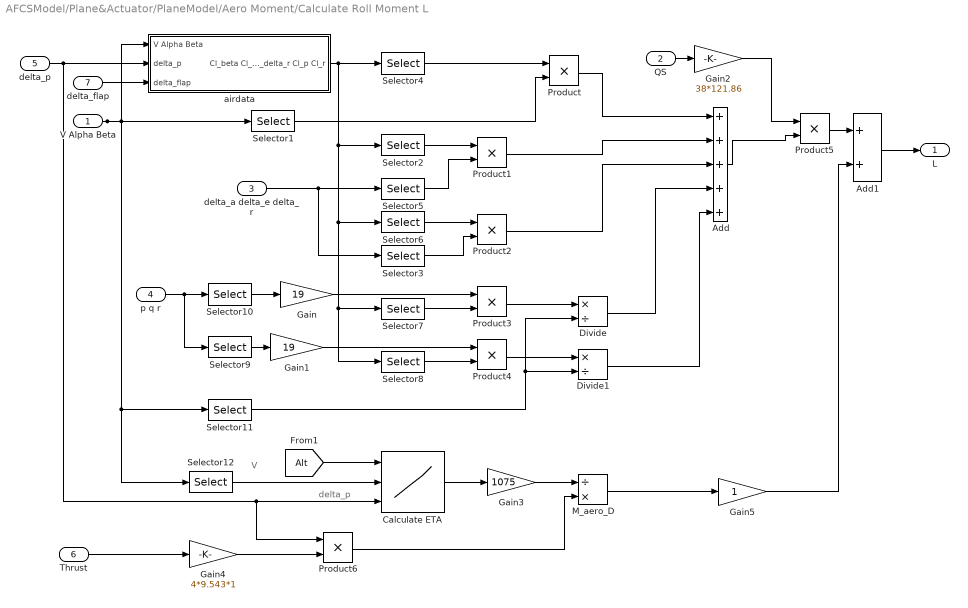
== system AFCSModel/Plane&Actuator/PlaneModel/Aero Moment/Calculate Roll Moment L ==
  note: V
  note: delta_p
  V Alpha Beta : Inport
  QS : Inport  Port=2
  delta_a delta_e delta_r : Inport  Port=3
  p q r : Inport  Port=4
  delta_p : Inport  Port=5
  Thrust : Inport  Port=6
  delta_flap : Inport  Port=7
  Add : Sum  Inputs=+++++
  Add1 : Sum
  Calculate ETA : Lookup_n-D  NumberOfTableDimensions=3  BreakpointsForDimension1=[0,1000,2000,3000,4000,5000,6000,7000,8000,9000,10000]  BreakpointsForDimension2=[50,100,150,175,200]  BreakpointsForDimension3=[0.4,0.6,0.7,0.85,1,1.04]  BreakpointsForDimension5=slselsubs({[1:3], [1:3], [1:3], [1:3], [1:3], [1:3], [1:3], [1:3], [1:3], [1:3], [1:3], [1:3], [1:3], [1:3], [1:3], [1:3], [1:3], [1:3], [1:3], [1:3], [1:3], [1:3], [1:3], [1:3], [1:3], [1:3]}, 1)  BreakpointsForDimension6=slselsubs({[1:3], [1:3], [1:3], [1:3], [1:3], [1:3], [1:3], [1:3], [1:3], [1:3], [1:3], [1:3], [1:3], [1:3], [1:3], [1:3], [1:3], [1:3], [1:3], [1:3], [1:3], [1:3], [1:3], [1:3], [1:3], [1:3]}, 2)  BreakpointsForDimension7=slselsubs({[1:3], [1:3], [1:3], [1:3], [1:3], [1:3], [1:3], [1:3], [1:3], [1:3], [1:3], [1:3], [1:3], [1:3], [1:3], [1:3], [1:3], [1:3], [1:3], [1:3], [1:3], [1:3], [1:3], [1:3], [1:3], [1:3]}, 3)  BreakpointsForDimension8=slselsubs({[1:3], [1:3], [1:3], [1:3], [1:3], [1:3], [1:3], [1:3], [1:3], [1:3], [1:3], [1:3], [1:3], [1:3], [1:3], [1:3], [1:3], [1:3], [1:3], [1:3], [1:3], [1:3], [1:3], [1:3], [1:3], [1:3]}, 4)  BreakpointsForDimension9=slselsubs({[1:3], [1:3], [1:3], [1:3], [1:3], [1:3], [1:3], [1:3], [1:3], [1:3], [1:3], [1:3], [1:3], [1:3], [1:3], [1:3], [1:3], [1:3], [1:3], [1:3], [1:3], [1:3], [1:3], [1:3], [1:3], [1:3]}, 5)  BreakpointsForDimension10=slselsubs({[1:3], [1:3], [1:3], [1:3], [1:3], [1:3], [1:3], [1:3], [1:3], [1:3], [1:3], [1:3], [1:3], [1:3], [1:3], [1:3], [1:3], [1:3], [1:3], [1:3], [1:3], [1:3], [1:3], [1:3], [1:3], [1:3]}, 6)  BreakpointsForDimension11=slselsubs({[1:3], [1:3], [1:3], [1:3], [1:3], [1:3], [1:3], [1:3], [1:3], [1:3], [1:3], [1:3], [1:3], [1:3], [1:3], [1:3], [1:3], [1:3], [1:3], [1:3], [1:3], [1:3], [1:3], [1:3], [1:3], [1:3]}, 7)  BreakpointsForDimension12=slselsubs({[1:3], [1:3], [1:3], [1:3], [1:3], [1:3], [1:3], [1:3], [1:3], [1:3], [1:3], [1:3], [1:3], [1:3], [1:3], [1:3], [1:3], [1:3], [1:3], [1:3], [1:3], [1:3], [1:3], [1:3], [1:3], [1:3]}, 8)  BreakpointsForDimension13=slselsubs({[1:3], [1:3], [1:3], [1:3], [1:3], [1:3], [1:3], [1:3], [1:3], [1:3], [1:3], [1:3], [1:3], [1:3], [1:3], [1:3], [1:3], [1:3], [1:3], [1:3], [1:3], [1:3], [1:3], [1:3], [1:3], [1:3]}, 9)  BreakpointsForDimension14=slselsubs({[1:3], [1:3], [1:3], [1:3], [1:3], [1:3], [1:3], [1:3], [1:3], [1:3], [1:3], [1:3], [1:3], [1:3], [1:3], [1:3], [1:3], [1:3], [1:3], [1:3], [1:3], [1:3], [1:3], [1:3], [1:3], [1:3]}, 10)  BreakpointsForDimension15=slselsubs({[1:3], [1:3], [1:3], [1:3], [1:3], [1:3], [1:3], [1:3], [1:3], [1:3], [1:3], [1:3], [1:3], [1:3], [1:3], [1:3], [1:3], [1:3], [1:3], [1:3], [1:3], [1:3], [1:3], [1:3], [1:3], [1:3]}, 11)  BreakpointsForDimension16=slselsubs({[1:3], [1:3], [1:3], [1:3], [1:3], [1:3], [1:3], [1:3], [1:3], [1:3], [1:3], [1:3], [1:3], [1:3], [1:3], [1:3], [1:3], [1:3], [1:3], [1:3], [1:3], [1:3], [1:3], [1:3], [1:3], [1:3]}, 12)  BreakpointsForDimension17=slselsubs({[1:3], [1:3], [1:3], [1:3], [1:3], [1:3], [1:3], [1:3], [1:3], [1:3], [1:3], [1:3], [1:3], [1:3], [1:3], [1:3], [1:3], [1:3], [1:3], [1:3], [1:3], [1:3], [1:3], [1:3], [1:3], [1:3]}, 13)  BreakpointsForDimension18=slselsubs({[1:3], [1:3], [1:3], [1:3], [1:3], [1:3], [1:3], [1:3], [1:3], [1:3], [1:3], [1:3], [1:3], [1:3], [1:3], [1:3], [1:3], [1:3], [1:3], [1:3], [1:3], [1:3], [1:3], [1:3], [1:3], [1:3]}, 14)  BreakpointsForDimension19=slselsubs({[1:3], [1:3], [1:3], [1:3], [1:3], [1:3], [1:3], [1:3], [1:3], [1:3], [1:3], [1:3], [1:3], [1:3], [1:3], [1:3], [1:3], [1:3], [1:3], [1:3], [1:3], [1:3], [1:3], [1:3], [1:3], [1:3]}, 15)  BreakpointsForDimension20=slselsubs({[1:3], [1:3], [1:3], [1:3], [1:3], [1:3], [1:3], [1:3], [1:3], [1:3], [1:3], [1:3], [1:3], [1:3], [1:3], [1:3], [1:3], [1:3], [1:3], [1:3], [1:3], [1:3], [1:3], [1:3], [1:3], [1:3]}, 16)  BreakpointsForDimension21=slselsubs({[1:3], [1:3], [1:3], [1:3], [1:3], [1:3], [1:3], [1:3], [1:3], [1:3], [1:3], [1:3], [1:3], [1:3], [1:3], [1:3], [1:3], [1:3], [1:3], [1:3], [1:3], [1:3], [1:3], [1:3], [1:3], [1:3]}, 17)  BreakpointsForDimension22=slselsubs({[1:3], [1:3], [1:3], [1:3], [1:3], [1:3], [1:3], [1:3], [1:3], [1:3], [1:3], [1:3], [1:3], [1:3], [1:3], [1:3], [1:3], [1:3], [1:3], [1:3], [1:3], [1:3], [1:3], [1:3], [1:3], [1:3]}, 18)  BreakpointsForDimension23=slselsubs({[1:3], [1:3], [1:3], [1:3], [1:3], [1:3], [1:3], [1:3], [1:3], [1:3], [1:3], [1:3], [1:3], [1:3], [1:3], [1:3], [1:3], [1:3], [1:3], [1:3], [1:3], [1:3], [1:3], [1:3], [1:3], [1:3]}, 19)  BreakpointsForDimension24=slselsubs({[1:3], [1:3], [1:3], [1:3], [1:3], [1:3], [1:3], [1:3], [1:3], [1:3], [1:3], [1:3], [1:3], [1:3], [1:3], [1:3], [1:3], [1:3], [1:3], [1:3], [1:3], [1:3], [1:3], [1:3], [1:3], [1:3]}, 20)  BreakpointsForDimension25=slselsubs({[1:3], [1:3], [1:3], [1:3], [1:3], [1:3], [1:3], [1:3], [1:3], [1:3], [1:3], [1:3], [1:3], [1:3], [1:3], [1:3], [1:3], [1:3], [1:3], [1:3], [1:3], [1:3], [1:3], [1:3], [1:3], [1:3]}, 21)  BreakpointsForDimension26=slselsubs({[1:3], [1:3], [1:3], [1:3], [1:3], [1:3], [1:3], [1:3], [1:3], [1:3], [1:3], [1:3], [1:3], [1:3], [1:3], [1:3], [1:3], [1:3], [1:3], [1:3], [1:3], [1:3], [1:3], [1:3], [1:3], [1:3]}, 22)  BreakpointsForDimension27=slselsubs({[1:3], [1:3], [1:3], [1:3], [1:3], [1:3], [1:3], [1:3], [1:3], [1:3], [1:3], [1:3], [1:3], [1:3], [1:3], [1:3], [1:3], [1:3], [1:3], [1:3], [1:3], [1:3], [1:3], [1:3], [1:3], [1:3]}, 23)  BreakpointsForDimension28=slselsubs({[1:3], [1:3], [1:3], [1:3], [1:3], [1:3], [1:3], [1:3], [1:3], [1:3], [1:3], [1:3], [1:3], [1:3], [1:3], [1:3], [1:3], [1:3], [1:3], [1:3], [1:3], [1:3], [1:3], [1:3], [1:3], [1:3]}, 24)  BreakpointsForDimension29=slselsubs({[1:3], [1:3], [1:3], [1:3], [1:3], [1:3], [1:3], [1:3], [1:3], [1:3], [1:3], [1:3], [1:3], [1:3], [1:3], [1:3], [1:3], [1:3], [1:3], [1:3], [1:3], [1:3], [1:3], [1:3], [1:3], [1:3]}, 25)  BreakpointsForDimension30=slselsubs({[1:3], [1:3], [1:3], [1:3], [1:3], [1:3], [1:3], [1:3], [1:3], [1:3], [1:3], [1:3], [1:3], [1:3], [1:3], [1:3], [1:3], [1:3], [1:3], [1:3], [1:3], [1:3], [1:3], [1:3], [1:3], [1:3]}, 26)  Table=ETA_data  InterpMethod=Cubic spline  ExtrapMethod=Cubic spline
      settings: InputPortMap=u0,u1,u2
  Divide : Product  Inputs=*/
  Divide1 : Product  Inputs=*/
  Gain : Gain  Gain=19
  Gain1 : Gain  Gain=19
  Gain2 : Gain  Gain=38*121.86
  Gain3 : Gain  Gain=1075
  Gain4 : Gain  Gain=4*9.543*1
  Gain5 : Gain
  M_aero_D : Product  Inputs=/*
  Product{,1..6} (7 alike) : Product  RndMeth=Zero
  Selector1 : Selector  InputPortWidth=3  IndexOptions=Index vector (dialog)  Indices=[3]  OutputSizes=[(-2)]
  Selector{5,10..12} (4 alike) : Selector  InputPortWidth=3  IndexOptions=Index vector (dialog)  Indices=[1]  OutputSizes=[(-2)]
  Selector2 : Selector  InputPortWidth=5  IndexOptions=Index vector (dialog)  Indices=[2]  OutputSizes=[(-2)]
  Selector3 : Selector  InputPortWidth=3  IndexOptions=Index vector (dialog)  Indices=[3]  OutputSizes=[(-2)]
  Selector4 : Selector  InputPortWidth=5  IndexOptions=Index vector (dialog)  Indices=[1]  OutputSizes=[(-2)]
  Selector6 : Selector  InputPortWidth=5  IndexOptions=Index vector (dialog)  Indices=[3]  OutputSizes=[(-2)]
  Selector7 : Selector  InputPortWidth=5  IndexOptions=Index vector (dialog)  Indices=[4]  OutputSizes=[(-2)]
  Selector8 : Selector  InputPortWidth=5  IndexOptions=Index vector (dialog)  Indices=[5]  OutputSizes=[(-2)]
  Selector9 : Selector  InputPortWidth=3  IndexOptions=Index vector (dialog)  Indices=[3]  OutputSizes=[(-2)]
  airdata : Subsystem
  L : Outport
  wires:
  airdata/1(Cl_beta Cl_delta_a Cl_delta_r Cl_p Cl_r) -> Selector4/1, Selector2/1, Selector6/1, Selector7/1, Selector8/1
  V Alpha Beta/1 -> Selector1/1, Selector11/1, Selector12/1, airdata/1(V Alpha Beta)
  Selector4/1 -> Product/1
  Selector1/1 -> Product/2
  Selector2/1 -> Product1/1
  delta_a delta_e delta_r/1 -> Selector5/1, Selector3/1
  Selector5/1 -> Product1/2
  Selector3/1 -> Product2/2
  Selector6/1 -> Product2/1
  p q r/1 -> Selector9/1, Selector10/1
  Selector9/1 -> Gain1/1
  Selector8/1 -> Product4/2
  Selector7/1 -> Product3/2
  Selector10/1 -> Gain/1
  Gain/1 -> Product3/1
  Gain1/1 -> Product4/1
  Selector11/1 -> Divide/2, Divide1/2
  Product4/1 -> Divide1/1
  Product3/1 -> Divide/1
  Product/1 -> Add/1
  Product1/1 -> Add/2
  Product2/1 -> Add/3
  Divide/1 -> Add/4
  Divide1/1 -> Add/5
  Add/1 -> Product5/2
  QS/1 -> Gain2/1
  Gain2/1 -> Product5/1
  delta_p/1 -> airdata/2(delta_p), Calculate ETA/3, Product6/1
  Product5/1 -> Add1/1
  Add1/1 -> L/1
  Calculate ETA/1 -> Gain3/1
  [Alt] -> Calculate ETA/1
  Selector12/1 -> Calculate ETA/2
  Gain3/1 -> M_aero_D/1
  Thrust/1 -> Gain4/1
  Gain4/1 -> Product6/2
  Product6/1 -> M_aero_D/2
  M_aero_D/1 -> Gain5/1
  Gain5/1 -> Add1/2
  delta_flap/1 -> airdata/3(delta_flap)

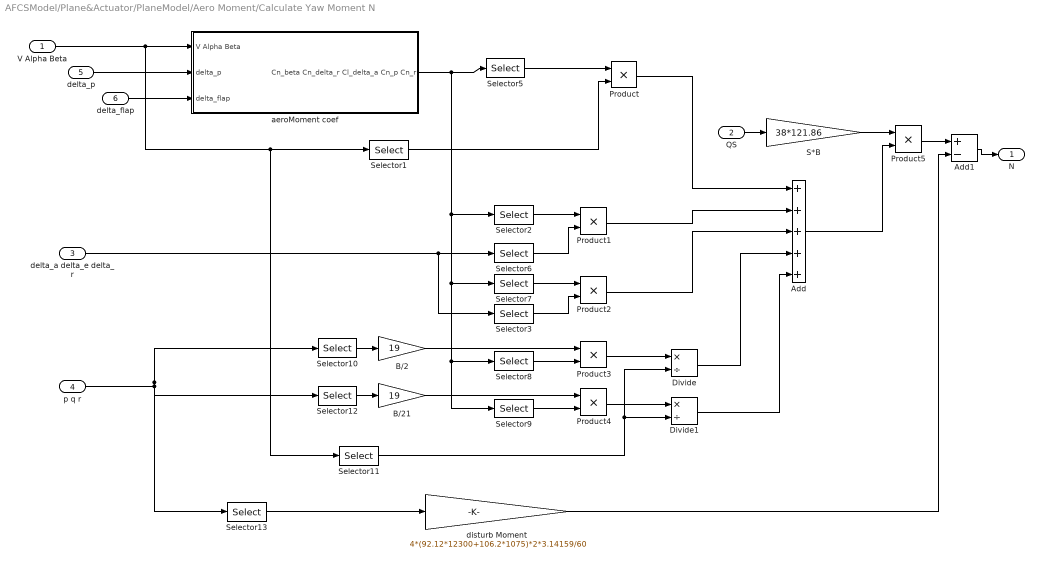
== system AFCSModel/Plane&Actuator/PlaneModel/Aero Moment/Calculate Yaw Moment N ==
  V Alpha Beta : Inport
  QS : Inport  Port=2
  delta_a delta_e delta_r : Inport  Port=3
  p q r : Inport  Port=4
  delta_p : Inport  Port=5
  delta_flap : Inport  Port=6
  Add : Sum  Inputs=+++++
  Add1 : Sum  Inputs=+-
  B/2 : Gain  Gain=19
  B/21 : Gain  Gain=19
  Divide : Product  Inputs=*/
  Divide1 : Product  Inputs=*/
  Product{,1..5} (6 alike) : Product  RndMeth=Zero
  S*B : Gain  Gain=38*121.86
  Selector1 : Selector  InputPortWidth=3  IndexOptions=Index vector (dialog)  Indices=[3]  OutputSizes=[(-2)]
  Selector10 : Selector  InputPortWidth=3  IndexOptions=Index vector (dialog)  Indices=[1]  OutputSizes=[(-2)]
  Selector11 : Selector  InputPortWidth=3  IndexOptions=Index vector (dialog)  Indices=[1]  OutputSizes=[(-2)]
  Selector12 : Selector  InputPortWidth=3  IndexOptions=Index vector (dialog)  Indices=[3]  OutputSizes=[(-2)]
  Selector13 : Selector  InputPortWidth=3  IndexOptions=Index vector (dialog)  Indices=[2]  OutputSizes=[(-2)]
  Selector2 : Selector  InputPortWidth=5  IndexOptions=Index vector (dialog)  Indices=[2]  OutputSizes=[(-2)]
  Selector3 : Selector  InputPortWidth=3  IndexOptions=Index vector (dialog)  Indices=[1]  OutputSizes=[(-2)]
  Selector5 : Selector  InputPortWidth=5  IndexOptions=Index vector (dialog)  Indices=[1]  OutputSizes=[(-2)]
  Selector6 : Selector  InputPortWidth=3  IndexOptions=Index vector (dialog)  Indices=[3]  OutputSizes=[(-2)]
  Selector7 : Selector  InputPortWidth=5  IndexOptions=Index vector (dialog)  Indices=[3]  OutputSizes=[(-2)]
  Selector8 : Selector  InputPortWidth=5  IndexOptions=Index vector (dialog)  Indices=[4]  OutputSizes=[(-2)]
  Selector9 : Selector  InputPortWidth=5  IndexOptions=Index vector (dialog)  Indices=[5]  OutputSizes=[(-2)]
  aeroMoment coef : Subsystem
  disturb Moment : Gain  Gain=4*(92.12*12300+106.2*1075)*2*3.14159/60
  N : Outport
  wires:
  V Alpha Beta/1 -> aeroMoment coef/1(V Alpha Beta), Selector1/1, Selector11/1
  delta_p/1 -> aeroMoment coef/2(delta_p)
  aeroMoment coef/1(Cn_beta Cn_delta_r Cl_delta_a Cn_p Cn_r) -> Selector5/1, Selector2/1, Selector7/1, Selector8/1, Selector9/1
  Selector5/1 -> Product/1
  Selector1/1 -> Product/2
  Selector2/1 -> Product1/1
  delta_a delta_e delta_r/1 -> Selector6/1, Selector3/1
  Selector6/1 -> Product1/2
  Selector3/1 -> Product2/2
  Selector7/1 -> Product2/1
  p q r/1 -> Selector12/1, Selector10/1, Selector13/1
  Selector12/1 -> B/21/1
  Selector9/1 -> Product4/2
  Selector8/1 -> Product3/2
  Selector10/1 -> B/2/1
  B/2/1 -> Product3/1
  B/21/1 -> Product4/1
  Selector11/1 -> Divide/2, Divide1/2
  Product4/1 -> Divide1/1
  Product3/1 -> Divide/1
  Product/1 -> Add/1
  Product1/1 -> Add/2
  Product2/1 -> Add/3
  Divide/1 -> Add/4
  Divide1/1 -> Add/5
  Add/1 -> Product5/2
  QS/1 -> S*B/1
  S*B/1 -> Product5/1
  Product5/1 -> Add1/1
  Add1/1 -> N/1
  Selector13/1 -> disturb Moment/1
  disturb Moment/1 -> Add1/2
  delta_flap/1 -> aeroMoment coef/3(delta_flap)
